simulink model "SimpleCtrl"  (R2020a)
settings: Solver=FixedStepDiscrete  StartTime=0.0  StopTime=0.4  RelTol=1e-3  EnableMultiTasking=on
InitFcn:
  | clc;
  | clear all;
  | 
  | lib_name = '';
  | 
  | if strcmp(computer, 'PCWIN')
  |   lib_name = 'dxl_x86_c';
  | elseif strcmp(computer, 'PCWIN64')
  |   lib_name = 'dxl_x64_c';
  | elseif strcmp(computer, 'GLNX86')
  |   lib_name = 'libdxl_x86_c';
  | elseif strcmp(computer, 'GLNXA64')
  |   lib_name = 'libdxl_x64_c';
  | elseif strcmp(computer, 'MACI64')
  |   lib_name = 'libdxl_mac_c';
  | end
  | 
  | % Load Libraries
  | if ~libisloaded(lib_name)
  |     [notfound, warnings] = loadlibrary(lib_name, 'dynamixel_sdk.h', 'addheader', 'port_handler.h', 'addheader', 'packet_handler.h');
  | end
  | 
  | % Control table address
  | ADDR_MX_TORQUE_ENABLE       = 24;           % Control table address is different in Dynamixel model
  | ADDR_MX_GOAL_POSITION       = 30;
  | ADDR_MX_PRESENT_POSITION    = 36;
  | 
  | % Protocol version
  | PROTOCOL_VERSION            = 1.0;          % See which protocol version is used in the Dynamixel
  | 
  | % Default setting
  | BAUDRATE                    = 1000000;
  | DEVICENAME                  = 'COM3';
  | 
  | TORQUE_ENABLE               = 1;            % Value for enabling the torque
  | TORQUE_DISABLE              = 0;            % Value for disabling the torque
  | DXL_MINIMUM_POSITION_VALUE  = 100;          % Dynamixel will rotate between this value
  | DXL_MAXIMUM_POSITION_VALUE  = 500;         % and this value (note that the Dynamixel would not move when the position value is out of movable range. Check e-manual about the range of the Dynamixel you use.)
  | DXL_MOVING_STATUS_THRESHOLD = 10;           % Dynamixel moving status threshold
  | 
  | COMM_SUCCESS                = 0;            % Communication Success result value
  | COMM_TX_FAIL                = -1001;        % Communication Tx Failed
  | Tstop = 8; % time at which Dynamixel motion is stopped
  | 
  | % Initialize PortHandler Structs
  | % Set the port path
  | % Get methods and members of PortHandlerLinux or PortHandlerWindows
  | port_num = portHandler(DEVICENAME);
  | 
  | % Initialize PacketHandler Structs
  | packetHandler();
  | 
  | dxl_comm_result = COMM_TX_FAIL;             % Communication result
  | 
  | dxl_error = 0;                              % Dynamixel error
  | dxl_present_position = 0;                   % Present position
  | 
  | 
  | % Open port
  | if (openPort(port_num))
  |     fprintf('Succeeded to open the port!\n');
  | else
  |     unloadlibrary(lib_name);
  |     fprintf('Failed to open the port!\n');
  |     input('Press any key to terminate...\n');
  |     dxl_error = 1000;
  |     return;
  | end
  | 
  | % Set port baudrate
  | if (setBaudRate(port_num, BAUDRATE))
  |     fprintf('Succeeded to change the baudrate!\n');
  | else
  |     unloadlibrary(lib_name);
  |     fprintf('Failed to change the baudrate!\n');
  |     input('Press any key to terminate...\n');
  |     dxl_error = 2000;
  |     return;
  | end
  | 
  | % set ID numbers of the the Dynamixels to be controlled:
  | ID01                     = 1;            % Dynamixel IDs for sagittal shoulders
  | ID02                     = 2;
  | ID03                     = 3;            % Dynamixel IDs for frontal shoulders
  | ID04                     = 4;
  | ID05                     = 5;            % Dynamixel IDs for elbows
  | ID06                     = 6;
  | ID07                     = 7;            % Dynamixel IDs for transverse hips
  | ID08                     = 8;
  | ID09                     = 9;            % Dynamixel IDs for frontal hips
  | ID10                     = 10;
  | ID11                     = 11;            % Dynamixel IDs for sagittal hips
  | ID12                     = 12;
  | ID13                     = 13;            % Dynamixel IDs for knees
  | ID14                     = 14;
  | ID15                     = 15;            % Dynamixel IDs for sagittal ankles
  | ID16                     = 16;
  | ID17                     = 17;            % Dynamixel IDs for frontal ankles
  | ID18                     = 18;
  | 
  | 
  | %% Enable Dynamixel Torques and connect Dynamixels
  | write1ByteTxRx(port_num, PROTOCOL_VERSION, ID01, ADDR_MX_TORQUE_ENABLE, TORQUE_ENABLE);
  | write1ByteTxRx(port_num, PROTOCOL_VERSION, ID02, ADDR_MX_TORQUE_ENABLE, TORQUE_ENABLE);
  | write1ByteTxRx(port_num, PROTOCOL_VERSION, ID03, ADDR_MX_TORQUE_ENABLE, TORQUE_ENABLE);
  | write1ByteTxRx(port_num, PROTOCOL_VERSION, ID04, ADDR_MX_TORQUE_ENABLE, TORQUE_ENABLE);
  | write1ByteTxRx(port_num, PROTOCOL_VERSION, ID05, ADDR_MX_TORQUE_ENABLE, TORQUE_ENABLE);
  | write1ByteTxRx(port_num, PROTOCOL_VERSION, ID06, ADDR_MX_TORQUE_ENABLE, TORQUE_ENABLE);
  | write1ByteTxRx(port_num, PROTOCOL_VERSION, ID07, ADDR_MX_TORQUE_ENABLE, TORQUE_ENABLE);
  | write1ByteTxRx(port_num, PROTOCOL_VERSION, ID08, ADDR_MX_TORQUE_ENABLE, TORQUE_ENABLE);
  | write1ByteTxRx(port_num, PROTOCOL_VERSION, ID09, ADDR_MX_TORQUE_ENABLE, TORQUE_ENABLE);
  | write1ByteTxRx(port_num, PROTOCOL_VERSION, ID10, ADDR_MX_TORQUE_ENABLE, TORQUE_ENABLE);
  | write1ByteTxRx(port_num, PROTOCOL_VERSION, ID11, ADDR_MX_TORQUE_ENABLE, TORQUE_ENABLE);
  | write1ByteTxRx(port_num, PROTOCOL_VERSION, ID12, ADDR_MX_TORQUE_ENABLE, TORQUE_ENABLE);
  | write1ByteTxRx(port_num, PROTOCOL_VERSION, ID13, ADDR_MX_TORQUE_ENABLE, TORQUE_ENABLE);
  | write1ByteTxRx(port_num, PROTOCOL_VERSION, ID14, ADDR_MX_TORQUE_ENABLE, TORQUE_ENABLE);
  | write1ByteTxRx(port_num, PROTOCOL_VERSION, ID15, ADDR_MX_TORQUE_ENABLE, TORQUE_ENABLE);
  | write1ByteTxRx(port_num, PROTOCOL_VERSION, ID16, ADDR_MX_TORQUE_ENABLE, TORQUE_ENABLE);
  | write1ByteTxRx(port_num, PROTOCOL_VERSION, ID17, ADDR_MX_TORQUE_ENABLE, TORQUE_ENABLE);
  | write1ByteTxRx(port_num, PROTOCOL_VERSION, ID18, ADDR_MX_TORQUE_ENABLE, TORQUE_ENABLE);
  | dxl_comm_result = getLastTxRxResult(port_num, PROTOCOL_VERSION);
  | dxl_error = getLastRxPacketError(port_num, PROTOCOL_VERSION);
  | if dxl_comm_result ~= COMM_SUCCESS
  |     fprintf('%s\n', getTxRxResult(PROTOCOL_VERSION, dxl_comm_result));
  | elseif dxl_error ~= 0
  |     fprintf('%s\n', getRxPacketError(PROTOCOL_VERSION, dxl_error));
  | else
  |     fprintf('Dynamixel has been successfully connected \n');
  | end
StopFcn:
  | %% Disable Dynamixel Torque and close program
  | write1ByteTxRx(port_num, PROTOCOL_VERSION, ID01, ADDR_MX_TORQUE_ENABLE, TORQUE_DISABLE);
  | write1ByteTxRx(port_num, PROTOCOL_VERSION, ID02, ADDR_MX_TORQUE_ENABLE, TORQUE_DISABLE);
  | write1ByteTxRx(port_num, PROTOCOL_VERSION, ID03, ADDR_MX_TORQUE_ENABLE, TORQUE_DISABLE);
  | write1ByteTxRx(port_num, PROTOCOL_VERSION, ID04, ADDR_MX_TORQUE_ENABLE, TORQUE_DISABLE);
  | write1ByteTxRx(port_num, PROTOCOL_VERSION, ID05, ADDR_MX_TORQUE_ENABLE, TORQUE_DISABLE);
  | write1ByteTxRx(port_num, PROTOCOL_VERSION, ID06, ADDR_MX_TORQUE_ENABLE, TORQUE_DISABLE);
  | write1ByteTxRx(port_num, PROTOCOL_VERSION, ID07, ADDR_MX_TORQUE_ENABLE, TORQUE_DISABLE);
  | write1ByteTxRx(port_num, PROTOCOL_VERSION, ID08, ADDR_MX_TORQUE_ENABLE, TORQUE_DISABLE);
  | write1ByteTxRx(port_num, PROTOCOL_VERSION, ID09, ADDR_MX_TORQUE_ENABLE, TORQUE_DISABLE);
  | write1ByteTxRx(port_num, PROTOCOL_VERSION, ID10, ADDR_MX_TORQUE_ENABLE, TORQUE_DISABLE);
  | write1ByteTxRx(port_num, PROTOCOL_VERSION, ID11, ADDR_MX_TORQUE_ENABLE, TORQUE_DISABLE);
  | write1ByteTxRx(port_num, PROTOCOL_VERSION, ID12, ADDR_MX_TORQUE_ENABLE, TORQUE_DISABLE);
  | write1ByteTxRx(port_num, PROTOCOL_VERSION, ID13, ADDR_MX_TORQUE_ENABLE, TORQUE_DISABLE);
  | write1ByteTxRx(port_num, PROTOCOL_VERSION, ID14, ADDR_MX_TORQUE_ENABLE, TORQUE_DISABLE);
  | write1ByteTxRx(port_num, PROTOCOL_VERSION, ID15, ADDR_MX_TORQUE_ENABLE, TORQUE_DISABLE);
  | write1ByteTxRx(port_num, PROTOCOL_VERSION, ID16, ADDR_MX_TORQUE_ENABLE, TORQUE_DISABLE);
  | write1ByteTxRx(port_num, PROTOCOL_VERSION, ID17, ADDR_MX_TORQUE_ENABLE, TORQUE_DISABLE);
  | write1ByteTxRx(port_num, PROTOCOL_VERSION, ID18, ADDR_MX_TORQUE_ENABLE, TORQUE_DISABLE);
  | dxl_comm_result = getLastTxRxResult(port_num, PROTOCOL_VERSION);
  | dxl_error = getLastRxPacketError(port_num, PROTOCOL_VERSION);
  |    if dxl_comm_result ~= COMM_SUCCESS
  |        fprintf('%s\n', getTxRxResult(PROTOCOL_VERSION, dxl_comm_result));
  |    elseif dxl_error ~= 0
  |        fprintf('%s\n', getRxPacketError(PROTOCOL_VERSION, dxl_error));
  |    end
  | 
  | % Close port
  | closePort(port_num);
  | 
  | % Unload Library
  | unloadlibrary(lib_name);
settings Model: SimulationMode=external  ExtModeTrigDuration=100  Creator=The MathWorks, Inc.  LastModifiedBy=JerryLee
settings SolverCC: PositivePriorityOrder=on
settings DataIOCC: LimitDataPoints=on  SaveFormat=Array  ReturnWorkspaceOutputs=off
settings OptimizationCC: ExpressionDepthLimit=2147483647  LifeSpan=Inf  MaxStackSize=64
settings DebuggingCC: UnderspecifiedInitializationDetection=Classic  MergeDetectMultiDrivingBlocksExec=none  FcnCallInpInsideContextMsg=warning  AllowSymbolicDim=off  StateNameClashWarn=warning  SFUnexpectedBacktrackingDiag=warning  SFNoUnconditionalDefaultTransitionDiag=warning  SFExecutionAtInitializationDiag=none  ArithmeticOperatorsInVariantConditions=warning
settings HardwareCC: ProdBitPerPointer=32  ProdBitPerSizeT=32  ProdBitPerPtrDiffT=32  ProdLargestAtomicInteger=Long  ProdLargestAtomicFloat=Double  ProdWordSize=32  ProdHWDeviceType=ARM Compatible->ARM Cortex  UseEmbeddedCoderFeatures=off  UseSimulinkCoderFeatures=off
settings ModelReferenceCC: PropagateSignalLabelsOutOfModel=off
settings SFSimCC: SimUseLocalCustomCode=off  MATLABDynamicMemAlloc=off  CustomCodeUndefinedFunction=UseInterfaceOnly
settings RTWCC: SystemTargetFile=ert.tlc  HardwareBoard=Raspberry Pi  TLCOptions=-aInlineSetEventsForThisBaseRateFcn=TLC_FALSE -aSuppressMultiTaskScheduler=TLC_FALSE -aRateBasedStepFcn=0  TemplateMakefile=ert_default_tmf  GenerateReport=on  RTWVerbose=off  RTWUseLocalCustomCode=off  Toolchain=GNU GCC Raspberry Pi  LaunchReport=on
settings CodeAppCC: ForceParamTrailComments=on  OperatorAnnotations=on  MangleLength=10  StateflowObjectComments=on  MATLABSourceComments=on
settings ERTTargetCC: MultiwordLength=2048  ERTCustomFileBanners=off  SupportContinuousTime=on  SupportNonInlinedSFcns=on  RemoveResetFunc=off  ModelStepFunctionPrototypeControlCompliant=off
settings ConfigComp: CovMetricSettings=dw  CovHtmlReporting=on  CovSaveCumulativeToWorkspaceVar=on  CovSaveSingleToWorkspaceVar=on  CovExternalEMLEnable=off

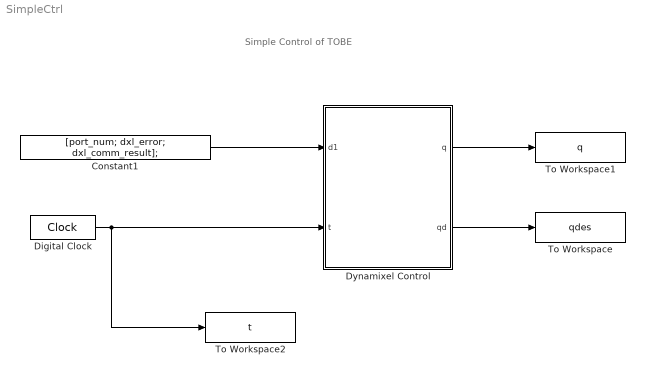
== system SimpleCtrl ==
  note: Simple Control of TOBE
  Constant1 : Constant  Value=[port_num; dxl_error; dxl_comm_result];
  Digital Clock : DigitalClock  SampleTime=0.01
  Dynamixel Control : MATLAB Function  TreatAsAtomicUnit=on
  To Workspace : ToWorkspace  VariableName=qdes  SampleTime=-1
  To Workspace1 : ToWorkspace  VariableName=q  SampleTime=-1
  To Workspace2 : ToWorkspace  VariableName=t  SampleTime=-1
  wires:
  Dynamixel Control/2(qd) -> To Workspace/1
  Dynamixel Control/1(q) -> To Workspace1/1
  Constant1/1 -> Dynamixel Control/1(d1)
  Digital Clock/1 -> To Workspace2/1, Dynamixel Control/2(t)

== matlab function SimpleCtrl/Dynamixel Control ==
  data: d1 input; q output; qd output; t input
function [q, qd] = runmotors(d1,t)
%#codegen
coder.extrinsic('write1ByteTxRx','write2ByteTxRx','read2ByteTxRx');
coder.extrinsic('getLastRxPacketError','getLastTxRxResult');
coder.extrinsic('getTxRxResult','getRxPacketError');
% coder.extrinsic('closePort','unloadlibrary');

% lib_name = 'dxl_x64_c';
port_num = d1(1);
dxl_error = d1(2);
dxl_comm_result = d1(3);

% Control table address
% ADDR_MX_TORQUE_ENABLE       = 24;           % Control table address is different in Dynamixel model
ADDR_MX_GOAL_POSITION       = 30;
ADDR_MX_PRESENT_POSITION    = 36;

% Protocol version
PROTOCOL_VERSION            = 1.0;          % See which protocol version is used in the Dynamixel

COMM_SUCCESS                = 0;            % Communication Success result value

%% Set Dynamixels and joint limits
% set ID numbers of the the Dynamixels to be controlled:
ID01                     = 1;            % Dynamixel IDs for sagittal shoulders
ID02                     = 2;
ID03                     = 3;            % Dynamixel IDs for frontal shoulders
ID04                     = 4;
ID05                     = 5;            % Dynamixel IDs for elbows
ID06                     = 6;
ID07                     = 7;            % Dynamixel IDs for transverse hips
ID08                     = 8;
ID09                     = 9;            % Dynamixel IDs for frontal hips
ID10                     = 10;
ID11                     = 11;            % Dynamixel IDs for sagittal hips
ID12                     = 12;
ID13                     = 13;            % Dynamixel IDs for knees
ID14                     = 14;
ID15                     = 15;            % Dynamixel IDs for sagittal ankles
ID16                     = 16;
ID17                     = 17;            % Dynamixel IDs for frontal ankles
ID18                     = 18;

% set joint limits
MIN01  = 0;            % right arm swung backward maximally
MID01  = 200;          % "home position" (arm down at side)
MAX01  = 500;          % arm swung out in front maximally

MIN02  = 500;          % left arm swung in front maximally
MID02  = 800;          % "home position" (arm down at side)
MAX02  = 1000;         % arm swung out backward maximally

MIN03  = 220;          % right upper arm swung inward maximally
MID03  = 300;          % "home position" 
MAX03  = 510;          % upper arm swung outward maximally 

MIN04  = 510;          % left upper arm swung outward maximally
MID04  = 720;          % "home position" 
MAX04  = 800;          % upper arm swung inward maximally

MIN05  = 230;          % right elbow bent maximally
MID05  = 450;          % "home position" 
MAX05  = 510;          % elbow extended maximally

MIN06  = 510;         % left elbow extended maximally 
MID06  = 570;         % "home position" 
MAX06  = 790;         % elbow bent maximally

MIN07  = 470;         % right leg turned inward maximally 
MID07  = 510;         % "home position" 
MAX07  = 550;         % leg turned outward maximally 

MIN08  = 470;         % left leg turned outward maximally 
MID08  = 510;         % "home position" 
MAX08  = 550;         % leg turned inward maximally

MIN09  = 490;          % right frontal hip swung inward maximally
MID09  = 510;          % "home position" 
MAX09  = 520;          % hip swung outward maximally (hard physical limit)

MIN10  = 500;          % left frontal hip swung outward maximally (hard physical limit)
MID10  = 510;          % "home position" 
MAX10  = 530;          % hip swung inward maximally

MIN11  = 300;          % right sagittal hip swung backward maximally
MID11  = 510;          % "home position" 
MAX11  = 850;          % hip swung forward maximally

MIN12  = 120;          % left sagittal hip swung forward maximally
MID12  = 510;          % "home position" 
MAX12  = 730;          % hip swung backward maximally

MIN13  = 220;          % right knee bent maximally
MID13  = 470;          % "home position" 
MAX13  = 510;          % knee extended maximally (hard physical limit)

MIN14  = 510;          % left knee extended maximally (hard physical limit)
MID14  = 550;          % "home position" 
MAX14  = 800;          % knee bent maximally

MIN15  = 400;          % right sagittal ankle, toes up maximally
MID15  = 510;          % "home position" 
MAX15  = 600;          % sagittal ankle, toes down maximally

MIN16  = 420;         % left sagittal ankle, toes down maximally 
MID16  = 510;         % "home position" 
MAX16  = 620;         % sagittal ankle, toes up maximally

MIN17  = 470;         % right frontal ankle turned up maximally (hard physical limit)
MID17  = 510;         % "home position" 
MAX17  = 600;         % frontal ankle turned down maximally 

MIN18  = 420;         % left frontal ankle turned down maximally 
MID18  = 510;         % "home position" 
MAX18  = 550;         % frontal ankle turned up maximally (hard physical limit)

interval = 0.02; 
index = mod(floor(t/interval),2)+1; % determine index of 1 or 2 based on time
time = mod(t,interval);

%% Set up goal position trajectories
GOAL01 = [MAX01,MIN01,MID01];                   % Goal positions for sagittal shoulders
GOAL02 = [MAX02,MIN02,MID02];
GOAL03 = [MAX03,MIN03,MID03];                   % Goal positions for frontal shoulders
GOAL04 = [MAX04,MIN04,MID04];
GOAL05 = [MAX05,MIN05,MID05];                   % Goal positions for elbows
GOAL06 = [MAX06,MIN06,MID06];
GOAL07 = [MAX07,MIN07,MID07];                   % Goal positions for transverse hips
GOAL08 = [MAX08,MIN08,MID08];
GOAL09 = [MAX09,MIN09,MID09];                   % Goal positions for frontal hips
GOAL10 = [MAX10,MIN10,MID10];
GOAL11 = [MAX11,MIN11,MID11];                   % Goal positions for sagittal hips
GOAL12 = [MAX12,MIN12,MID12];
GOAL13 = [MAX13,MIN13,MID13];                   % Goal positions for knees
GOAL14 = [MIN14,MAX14,MID14];
GOAL15 = [MAX15,MIN15,MID15];                   % Goal positions for sagittal ankles
GOAL16 = [MAX16,MIN16,MID16];
GOAL17 = [MAX17,MIN17,MID17];                   % Goal positions for frontal ankles
GOAL18 = [MAX18,MIN18,MID18];

%% Set command positions for joints at constant position
    CMD01 = 0.5*(300-100)*cos((pi/interval)*(time + interval*(index-1))) + 0.5*(300+100); %GOAL01(ind1);
    CMD02 = 0.5*(900-700)*cos((pi/interval)*(time + interval*(index-1))) + 0.5*(900+700); %GOAL02(ind1);
    CMD03 = GOAL03(3); 
    CMD04 = GOAL04(3);
    CMD05 = GOAL05(2);
    CMD06 = GOAL06(1);   
    CMD07 = GOAL07(3);   
    CMD08 = GOAL08(3);    
    CMD09 = GOAL09(1); 
    CMD10 = GOAL10(2);   
    CMD11 = 0.5*(MIN11-MAX11)*cos((pi/interval)*(time + interval*(index-1))) + 0.5*(MAX11+MIN11); %GOAL11(ind1);
    CMD12 = 0.5*(MIN12-MAX12)*cos((pi/interval)*(time + interval*(index-1))) + 0.5*(MAX12+MIN12); %GOAL12(ind1); 
    CMD13 = 0.5*(MIN13-MAX13)*cos((2*pi/interval)*time) + 0.5*(MAX13+MIN13); %GOAL13(index); 
    CMD14 = 0.5*(MAX14-MIN14)*cos((2*pi/interval)*time) + 0.5*(MAX14+MIN14); %GOAL14(index);
    CMD15 = GOAL15(3);
    CMD16 = GOAL16(3);   
    CMD17 = GOAL17(2);   
    CMD18 = GOAL18(1); 

%% Send command positions to motors
    write2ByteTxRx(port_num, PROTOCOL_VERSION, ID01, ADDR_MX_GOAL_POSITION, CMD01);
    write2ByteTxRx(port_num, PROTOCOL_VERSION, ID02, ADDR_MX_GOAL_POSITION, CMD02);
    write2ByteTxRx(port_num, PROTOCOL_VERSION, ID03, ADDR_MX_GOAL_POSITION, CMD03);
    write2ByteTxRx(port_num, PROTOCOL_VERSION, ID04, ADDR_MX_GOAL_POSITION, CMD04);
    write2ByteTxRx(port_num, PROTOCOL_VERSION, ID05, ADDR_MX_GOAL_POSITION, CMD05);
    write2ByteTxRx(port_num, PROTOCOL_VERSION, ID06, ADDR_MX_GOAL_POSITION, CMD06);
    write2ByteTxRx(port_num, PROTOCOL_VERSION, ID07, ADDR_MX_GOAL_POSITION, CMD07);
    write2ByteTxRx(port_num, PROTOCOL_VERSION, ID08, ADDR_MX_GOAL_POSITION, CMD08);
    write2ByteTxRx(port_num, PROTOCOL_VERSION, ID09, ADDR_MX_GOAL_POSITION, CMD09);
    write2ByteTxRx(port_num, PROTOCOL_VERSION, ID10, ADDR_MX_GOAL_POSITION, CMD10);
    write2ByteTxRx(port_num, PROTOCOL_VERSION, ID11, ADDR_MX_GOAL_POSITION, CMD11);
    write2ByteTxRx(port_num, PROTOCOL_VERSION, ID12, ADDR_MX_GOAL_POSITION, CMD12);
    write2ByteTxRx(port_num, PROTOCOL_VERSION, ID13, ADDR_MX_GOAL_POSITION, CMD13);
    write2ByteTxRx(port_num, PROTOCOL_VERSION, ID14, ADDR_MX_GOAL_POSITION, CMD14);
    write2ByteTxRx(port_num, PROTOCOL_VERSION, ID15, ADDR_MX_GOAL_POSITION, CMD15);
    write2ByteTxRx(port_num, PROTOCOL_VERSION, ID16, ADDR_MX_GOAL_POSITION, CMD16);
    write2ByteTxRx(port_num, PROTOCOL_VERSION, ID17, ADDR_MX_GOAL_POSITION, CMD17);
    write2ByteTxRx(port_num, PROTOCOL_VERSION, ID18, ADDR_MX_GOAL_POSITION, CMD18);
    
dxl_comm_result = getLastTxRxResult(port_num, PROTOCOL_VERSION);
dxl_error = getLastRxPacketError(port_num, PROTOCOL_VERSION);
if dxl_comm_result ~= COMM_SUCCESS
    fprintf('%s\n', getTxRxResult(PROTOCOL_VERSION, dxl_comm_result));
elseif dxl_error ~= 0
    fprintf('%s\n', getRxPacketError(PROTOCOL_VERSION, dxl_error));
end

%% Read present position
    NOW01 = read2ByteTxRx(port_num, PROTOCOL_VERSION, ID01, ADDR_MX_PRESENT_POSITION);
    NOW02 = read2ByteTxRx(port_num, PROTOCOL_VERSION, ID02, ADDR_MX_PRESENT_POSITION);
    NOW03 = read2ByteTxRx(port_num, PROTOCOL_VERSION, ID03, ADDR_MX_PRESENT_POSITION);
    NOW04 = read2ByteTxRx(port_num, PROTOCOL_VERSION, ID04, ADDR_MX_PRESENT_POSITION);
    NOW05 = read2ByteTxRx(port_num, PROTOCOL_VERSION, ID05, ADDR_MX_PRESENT_POSITION);
    NOW06 = read2ByteTxRx(port_num, PROTOCOL_VERSION, ID06, ADDR_MX_PRESENT_POSITION);
    NOW07 = read2ByteTxRx(port_num, PROTOCOL_VERSION, ID07, ADDR_MX_PRESENT_POSITION);
    NOW08 = read2ByteTxRx(port_num, PROTOCOL_VERSION, ID08, ADDR_MX_PRESENT_POSITION);
    NOW09 = read2ByteTxRx(port_num, PROTOCOL_VERSION, ID09, ADDR_MX_PRESENT_POSITION);
    NOW10 = read2ByteTxRx(port_num, PROTOCOL_VERSION, ID10, ADDR_MX_PRESENT_POSITION);
    NOW11 = read2ByteTxRx(port_num, PROTOCOL_VERSION, ID11, ADDR_MX_PRESENT_POSITION);
    NOW12 = read2ByteTxRx(port_num, PROTOCOL_VERSION, ID12, ADDR_MX_PRESENT_POSITION);
    NOW13 = read2ByteTxRx(port_num, PROTOCOL_VERSION, ID13, ADDR_MX_PRESENT_POSITION);
    NOW14 = read2ByteTxRx(port_num, PROTOCOL_VERSION, ID14, ADDR_MX_PRESENT_POSITION);
    NOW15 = read2ByteTxRx(port_num, PROTOCOL_VERSION, ID15, ADDR_MX_PRESENT_POSITION);
    NOW16 = read2ByteTxRx(port_num, PROTOCOL_VERSION, ID16, ADDR_MX_PRESENT_POSITION);
    NOW17 = read2ByteTxRx(port_num, PROTOCOL_VERSION, ID17, ADDR_MX_PRESENT_POSITION);
    NOW18 = read2ByteTxRx(port_num, PROTOCOL_VERSION, ID18, ADDR_MX_PRESENT_POSITION);
dxl_comm_result = getLastTxRxResult(port_num, PROTOCOL_VERSION);
dxl_error = getLastRxPacketError(port_num, PROTOCOL_VERSION);

if dxl_comm_result ~= COMM_SUCCESS
    fprintf('%s\n', getTxRxResult(PROTOCOL_VERSION, dxl_comm_result));
elseif dxl_error ~= 0
    fprintf('%s\n', getRxPacketError(PROTOCOL_VERSION, dxl_error));
end

%     fprintf('[ID:%03d] CmdPos:%03d  PresPos:%03d\n', ID01, CMD01, NOW01);
%     fprintf('[ID:%03d] CmdPos:%03d  PresPos:%03d\n', ID02, CMD02, NOW02);
%     fprintf('[ID:%03d] CmdPos:%03d  PresPos:%03d\n', ID03, CMD03, NOW03);
%     fprintf('[ID:%03d] CmdPos:%03d  PresPos:%03d\n', ID04, CMD04, NOW04);
%     fprintf('[ID:%03d] CmdPos:%03d  PresPos:%03d\n', ID05, CMD05, NOW05);
%     fprintf('[ID:%03d] CmdPos:%03d  PresPos:%03d\n', ID06, CMD06, NOW06);
%     fprintf('[ID:%03d] CmdPos:%03d  PresPos:%03d\n', ID07, CMD07, NOW07);
%     fprintf('[ID:%03d] CmdPos:%03d  PresPos:%03d\n', ID08, CMD08, NOW08);
%     fprintf('[ID:%03d] CmdPos:%03d  PresPos:%03d\n', ID09, CMD09, NOW09);
%     fprintf('[ID:%03d] CmdPos:%03d  PresPos:%03d\n', ID10, CMD10, NOW10);
%     fprintf('[ID:%03d] CmdPos:%03d  PresPos:%03d\n', ID11, CMD11, NOW11);
%     fprintf('[ID:%03d] CmdPos:%03d  PresPos:%03d\n', ID12, CMD12, NOW12);        
%     fprintf('[ID:%03d] CmdPos:%03d  PresPos:%03d\n', ID13, CMD13, NOW13);
%     fprintf('[ID:%03d] CmdPos:%03d  PresPos:%03d\n', ID14, CMD14, NOW14);
%     fprintf('[ID:%03d] CmdPos:%03d  PresPos:%03d\n', ID15, CMD15, NOW15);
%     fprintf('[ID:%03d] CmdPos:%03d  PresPos:%03d\n', ID16, CMD16, NOW16);
%     fprintf('[ID:%03d] CmdPos:%03d  PresPos:%03d\n', ID17, CMD17, NOW17);
%     fprintf('[ID:%03d] CmdPos:%03d  PresPos:%03d\n', ID18, CMD18, NOW18);
    
% the following two lines seem unnecessary, 
% but don't delete them, or it will throw an error:
q = zeros(18,1);
qd = zeros(18,1);

q = [NOW01;NOW02;NOW03;NOW04;NOW05;NOW06;NOW07;NOW08;NOW09;NOW10;NOW11;NOW12;NOW13;NOW14;NOW15;NOW16;NOW17;NOW18];
qd = [CMD01;CMD02;CMD03;CMD04;CMD05;CMD06;CMD07;CMD08;CMD09;CMD10;CMD11;CMD12;CMD13;CMD14;CMD15;CMD16;CMD17;CMD18];
